simulink model "Bat_SPM"  (R2024a)
settings: Solver=FixedStepAuto  StartTime=0.0  StopTime=t_end  FixedStep=dt  MaxStep=dt  RelTol=1e-3  EnableMultiTasking=on
values from neighbouring files (symbols this model uses):
  I = squeeze(out.I.Data)./4.6    [PI_init.m]
  P0 = 4.1374e3    (= 4137.4)    [PI_init.m]
  Params_P = [sig0,P_atm,E,alpha_cell,Tamb,L,Vh0,A_surf,m_an,xSEI0,MC6,R,A1,B1,     C1,A2,B2,C2,yEC,yDMC]    [PI_init.m]
  V_min = 0    [PI_init.m]
libraries: slpidlib x1
settings Model: Creator=imanebrahimi  LastModifiedBy=imanebrahimi
settings SolverCC: AutoInsertRateTranBlk=on
settings OptimizationCC: DefaultParameterBehavior=Inlined  InlineInvariantSignals=on  EnhancedBackFolding=on  PassReuseOutputArgsAs=Individual arguments  StateBitsets=on  DataBitsets=on  ZeroExternalMemoryAtStartup=off  ZeroInternalMemoryAtStartup=off  NoFixptDivByZeroProtection=on  LifeSpan=1  OptimizeBlockOrder=speed  DifferentSizesBufferReuse=on  EfficientTunableParamExpr=on
settings DebuggingCC: ParameterTunabilityLossMsg=error
settings HardwareCC: ProdBitPerPointer=32  ProdBitPerSizeT=32  ProdBitPerPtrDiffT=32  ProdLargestAtomicFloat=None  ProdIntDivRoundTo=Floor  ProdWordSize=32  ProdHWDeviceType=Generic->Custom
settings SFSimCC: MATLABDynamicMemAlloc=off
settings RTWCC: Description=Embedded Coder  SystemTargetFile=ert.tlc  TLCOptions=-p0  GenCodeOnly=on  TemplateMakefile=ert_default_tmf  GenerateReport=on  RTWVerbose=off  IncludeHyperlinkInReport=on  LaunchReport=on  GPUComputeCapability=3.5
settings CodeAppCC: ForceParamTrailComments=on  IgnoreCustomStorageClasses=off  OperatorAnnotations=on  SimulinkDataObjDesc=on  SFDataObjDesc=on  CustomSymbolStrGlobalVar=rt$N$M  CustomSymbolStrType=$N$M  CustomSymbolStrFcn=$N$M$F  CustomSymbolStrMacro=$N$M  InsertBlockDesc=on
settings ERTTargetCC: TargetLangStandard=C99 (ISO)  CodeReplacementLibrary=ISO_C  GenerateSampleERTMain=on  IncludeMdlTerminateFcn=off  SuppressErrorStatus=on  SupportAbsoluteTime=off  PurelyIntegerCode=on  SupportNonFinite=off  SupportComplex=off  InlinedParameterPlacement=NonHierarchical  RootIOFormat=Structure reference  ERTCustomFileTemplate=example_file_process.tlc

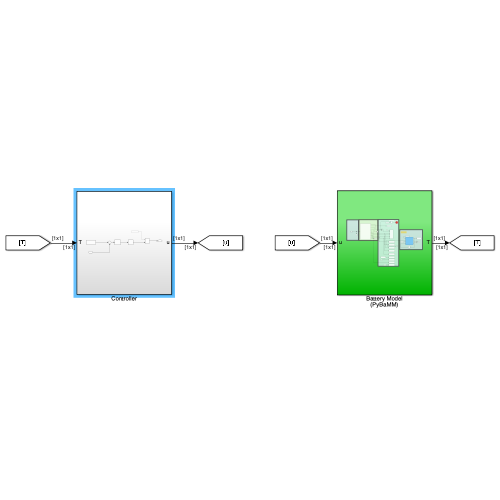
[thumbnail: Simulink's stored preview of the top-level diagram]
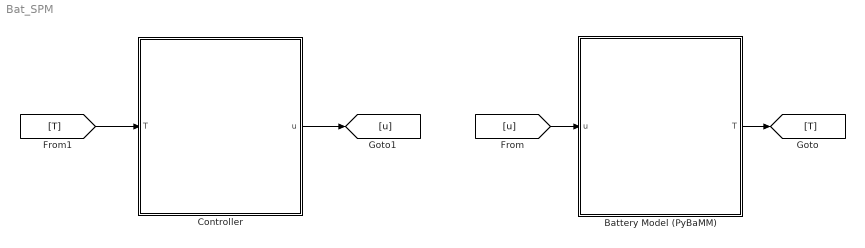
== system Bat_SPM ==
  Battery Model (PyBaMM) : Subsystem
  Controller : Subsystem
  wires:
  [u] -> Battery Model (PyBaMM)/1(u)
  [T] -> Controller/1(T)
  Controller/1(u) -> [u]
  Battery Model (PyBaMM)/1(T) -> [T]

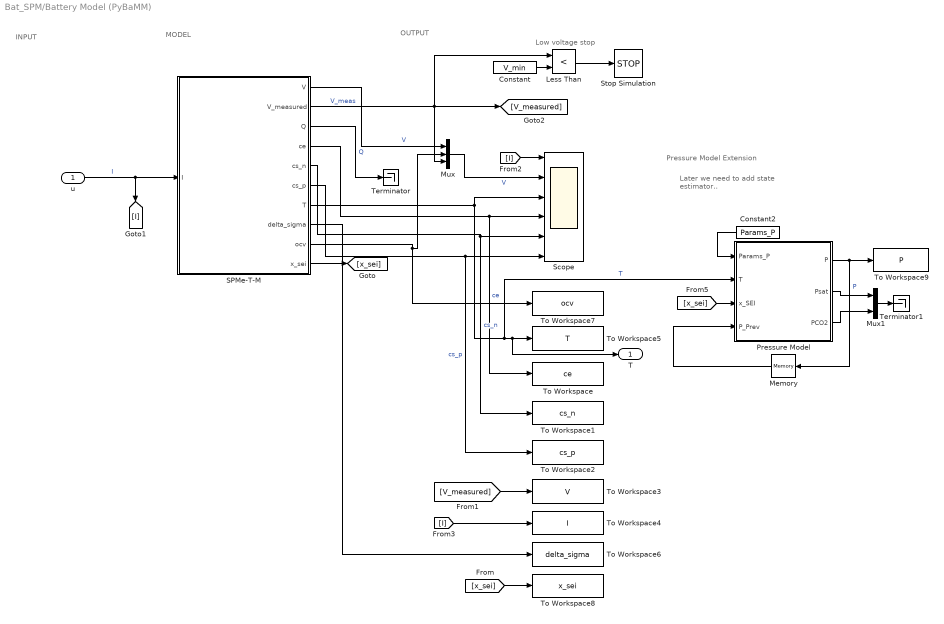
== system Bat_SPM/Battery Model (PyBaMM) ==
  note: INPUT
  note: Low voltage stop
  note: OUTPUT
  note: MODEL
  note: Later we need to add state estimator..
  note: Pressure Model Extension
  u : Inport
  Constant : Constant  Value=V_min
  Constant2 : Constant  Value=Params_P
  Less Than : RelationalOperator  Operator=<  OutDataTypeStr=boolean  RndMeth=Simplest  InputSameDT=off
  Memory : Memory  InitialCondition=P0  InheritSampleTime=on  LinearizeAsDelay=on
  Mux : Mux  Inputs=3
  Mux1 : Mux  Inputs=2
  Pressure Model : MATLAB Function  TreatAsAtomicUnit=on
  SPMe-T-M : Subsystem
  Scope : Scope  NumInputPorts=6
  Stop Simulation : Stop
  Terminator : Terminator
  Terminator1 : Terminator
  To Workspace : ToWorkspace  VariableName=ce  SaveFormat=Timeseries  SampleTime=-1
  To Workspace1 : ToWorkspace  VariableName=cs_n  SaveFormat=Timeseries  SampleTime=-1
  To Workspace2 : ToWorkspace  VariableName=cs_p  SaveFormat=Timeseries  SampleTime=-1
  To Workspace3 : ToWorkspace  VariableName=V  SaveFormat=Timeseries  SampleTime=-1
  To Workspace4 : ToWorkspace  VariableName=I  SaveFormat=Timeseries  SampleTime=-1
  To Workspace5 : ToWorkspace  VariableName=T  SaveFormat=Timeseries  SampleTime=-1
  To Workspace6 : ToWorkspace  VariableName=delta_sigma  SaveFormat=Timeseries  SampleTime=-1
  To Workspace7 : ToWorkspace  VariableName=ocv  SaveFormat=Timeseries  SampleTime=-1
  To Workspace8 : ToWorkspace  VariableName=x_sei  SaveFormat=Timeseries  SampleTime=-1
  To Workspace9 : ToWorkspace  VariableName=P  SaveFormat=Timeseries  SampleTime=-1
  T : Outport
  wires:
  SPMe-T-M/2(V_measured) -> Less Than/1, Mux/3, [V_measured]  "V_meas"
  [V_measured] -> To Workspace3/1
  SPMe-T-M/6(cs_p) -> To Workspace2/1, Scope/6  "cs_p"
  Mux/1 -> Scope/2  "V"
  Less Than/1 -> Stop Simulation/1
  [I] -> Scope/1
  SPMe-T-M/5(cs_n) -> To Workspace1/1, Scope/5  "cs_n"
  Constant/1 -> Less Than/2
  [I] -> To Workspace4/1
  SPMe-T-M/9(ocv) -> Mux/2, To Workspace7/1
  SPMe-T-M/3(Q) -> Terminator/1  "Q"
  SPMe-T-M/1(V) -> Mux/1  "V"
  u/1 -> SPMe-T-M/1(I), [I]  "I"
  SPMe-T-M/8(delta_sigma) -> To Workspace6/1
  SPMe-T-M/7(T) -> Pressure Model/2(T), T/1, To Workspace5/1, Scope/3  "T"
  SPMe-T-M/4(ce) -> To Workspace/1, Scope/4  "ce"
  SPMe-T-M/10(x_sei) -> [x_sei]
  [x_sei] -> To Workspace8/1
  Pressure Model/2(Psat) -> Mux1/1
  Mux1/1 -> Terminator1/1
  Pressure Model/3(PCO2) -> Mux1/2
  Pressure Model/1(P) -> To Workspace9/1, Memory/1  "P"
  Memory/1 -> Pressure Model/4(P_Prev)
  Constant2/1 -> Pressure Model/1(Params_P)
  [x_sei] -> Pressure Model/3(x_SEI)

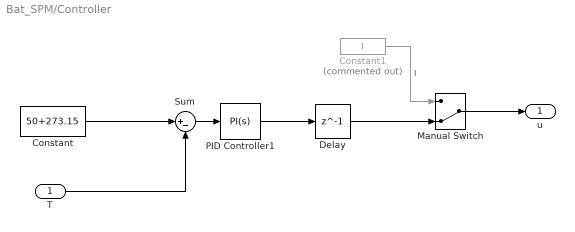
== system Bat_SPM/Controller ==
  T : Inport
  Constant : Constant  Value=50+273.15
  Constant1 : Constant  Commented=on  Value=I
  Delay : Delay  DelayLength=1
  Manual Switch : ManualSwitch  CurrentSetting=0
  PID Controller1 : slpidlib/PID Controller  Controller=PI  Form=Parallel  TimeDomain=Continuous-time  UseExternalTs=off  SampleTime=-1  IntegratorMethod=Forward Euler  FilterMethod=Forward Euler  ControllerParametersSource=internal  P=7.95363343093835  I=0.0486588718627495  UseKiTs=off  D=0  UseExternalDerivativeSource=off  N=100  UseFilter=on  TunerSelectOption=Transfer Function Based (PID Tuner App)  InitialConditionSource=internal  InitialConditionForIntegrator=0  InitialConditionForFilter=0  DifferentiatorICPrevScaledInput=0  ExternalReset=none  TrackingMode=off  Kt=1  LimitOutput=off  SatLimitsSource=internal  UpperSaturationLimit=46  LowerSaturationLimit=0  LinearizeAsGain=on  AntiWindupMode=none  Kb=1  LimitIntegrator=off  UpperIntegratorSaturationLimit=inf  LowerIntegratorSaturationLimit=-inf  POutMin=[]  POutMax=[]  IOutMin=[]  IOutMax=[]  DOutMin=[]  DOutMax=[]  NOutMin=[]  NOutMax=[]  SumOutMin=[]  SumOutMax=[]  SaturationOutMin=[]  SaturationOutMax=[]  PParamMin=[]  PParamMax=[]  IParamMin=[]  IParamMax=[]  DParamMin=[]  DParamMax=[]  NParamMin=[]  NParamMax=[]  KbParamMin=[]  KbParamMax=[]  KtParamMin=[]  KtParamMax=[]  KbOutMin=[]  KbOutMax=[]  KtOutMin=[]  KtOutMax=[]  IntegratorOutMin=[]  IntegratorOutMax=[]  FilterOutMin=[]  FilterOutMax=[]  SumI1OutMin=[]  SumI1OutMax=[]  SumI2OutMin=[]  SumI2OutMax=[]  SumI3OutMin=[]  SumI3OutMax=[]  SumI4OutMin=[]  SumI4OutMax=[]  SumDOutMin=[]  SumDOutMax=[]  DifferentiatorOutMin=[]  DifferentiatorOutMax=[]  FilterDiffOutCoefMin=[]  FilterDiffOutCoefMax=[]  ReciprocalOutMin=[]  ReciprocalOutMax=[]  SumDenOutMin=[]  SumDenOutMax=[]  SumNumOutMin=[]  SumNumOutMax=[]  DivideOutMin=[]  DivideOutMax=[]  UdiffTsProdOutMin=[]  UdiffTsProdOutMax=[]  NTsProdOutMin=[]  NTsProdOutMax=[]  UintegralTsProdOutMin=[]  UintegralTsProdOutMax=[]  UngainTsProdOutMin=[]  UngainTsProdOutMax=[]  ClampingZeroOutDataTypeStr=Inherit: Inherit via back propagation  ClampingZeroOutMin=[]  ClampingZeroOutMax=[]  FilterDenConstantOutDataTypeStr=Inherit: Inherit via back propagation  FilterDenConstantOutMin=[]  FilterDenConstantOutMax=[]  PCopyOutDataTypeStr=Inherit: Inherit via back propagation  PCopyOutMin=[]  PCopyOutMax=[]  NCopyOutDataTypeStr=Inherit: Inherit via back propagation  NCopyOutMin=[]  NCopyOutMax=[]  IntegratorContinuousStateAttributes=''  IntegratorStateMustResolveToSignalObject=off  IntegratorRTWStateStorageClass=Auto  FilterContinuousStateAttributes=''  FilterStateMustResolveToSignalObject=off  FilterRTWStateStorageClass=Auto  ParallelPVariant=InternalParameters  IdealPVariant=Disabled  IVariant=InternalParameters  DVariant=Disabled  IntegratorVariant=Continuous  SatVariant=Disabled  AWVariant=Passthrough  PCopyVariant=Disabled  TRVariant=Disabled  FdbkBlocksVariant=Forward  IdealPFdbkVariant=Disabled  SatFdbkVariant=Disabled  DerivativeFilterVariant=Disabled  NVariant=Disabled  NCopyVariant=Disabled_SignalSpec  FilterICVariant=Disabled  IntegratorICVariant=InternalICs  ExternalResetVariant=Disabled  TRSumVariant=Passthrough  SumFdbkVariant=Disabled  SumVariant=Sum_PI  TsampFilterVariant=InternalTs  TsampNgainVariant=Passthrough  TsampIntegralVariant=Disabled_SignalSpec  ExternalSaturationOutDataTypeStr=Inherit: Same as second input  DerivativeSourceVariant=Disabled
  Sum : Sum  Inputs=|+-
  u : Outport
  wires:
  Manual Switch/1 -> u/1
  Sum/1 -> PID Controller1/1
  PID Controller1/1 -> Delay/1
  Constant/1 -> Sum/1
  Constant1/1 -> Manual Switch/1  "I"
  Delay/1 -> Manual Switch/2
  T/1 -> Sum/2

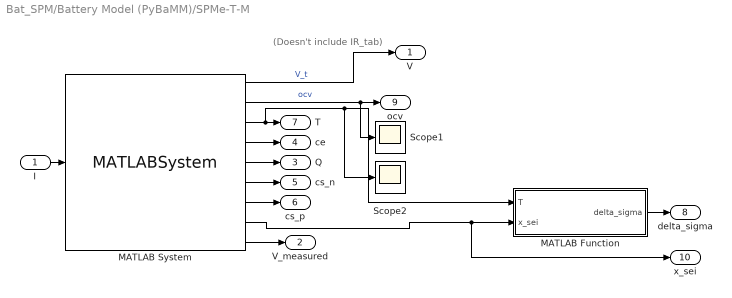
== system Bat_SPM/Battery Model (PyBaMM)/SPMe-T-M ==
  note: (Doesn't include IR_tab)
  I : Inport
  MATLAB Function : MATLAB Function  TreatAsAtomicUnit=on
  MATLAB System : MATLABSystem  System=pybamm_bat  SimulateUsing=Interpreted execution
      mask Type: pybamm_bat
      mask Display:
      | disp('pybamm_bat');
      | port_label('input',1,'current');
      | port_label('output',1,'V_t');
      | port_label('output',2,'ocv');
      | port_label('output',3,'T');
      | port_label('output',4,'ce');
      | port_label('output',5,'heating');
      | port_label('output',6,'neg_conc');
      | port_label('output',7,'pos_conc');
      | port_label('output',8,'x_sei');
      | port_label('output',9,'V_meas');
  Scope1 : Scope
  Scope2 : Scope
  V : Outport
  V_measured : Outport  Port=2
  Q : Outport  Port=3  VectorParamsAs1DForOutWhenUnconnected=off
  ce : Outport  Port=4
  cs_n : Outport  Port=5  VectorParamsAs1DForOutWhenUnconnected=off
  cs_p : Outport  Port=6  VectorParamsAs1DForOutWhenUnconnected=off
  T : Outport  Port=7
  delta_sigma : Outport  Port=8
  ocv : Outport  Port=9
  x_sei : Outport  Port=10
  wires:
  MATLAB System/4 -> ce/1
  MATLAB System/5 -> Q/1
  MATLAB System/6 -> cs_n/1
  MATLAB System/7 -> cs_p/1
  MATLAB System/1 -> V/1  "V_t"
  MATLAB System/9 -> V_measured/1
  MATLAB System/2 -> Scope1/1, ocv/1  "ocv"
  I/1 -> MATLAB System/1
  MATLAB System/3 -> MATLAB Function/1(T), Scope2/1, T/1
  MATLAB System/8 -> x_sei/1, MATLAB Function/2(x_sei)
  MATLAB Function/1(delta_sigma) -> delta_sigma/1

== matlab function Bat_SPM/Battery Model (PyBaMM)/SPMe-T-M/MATLAB Function ==
  data: T input; x_sei input; delta_sigma output
function delta_sigma  = expansion(T,x_sei)
%XSEI2PTOTAL 
% Mechanical params
M_C6 = 72/1000; %kg/mol
% V_head_0 = 6.65e-6; %m3 (0.121*0.074*0.0055)*0.135
% L = 2.4/1000; %m
% E = 0.19e6; %Pa
% alpha_cell = 1.1e-6; %m/K
% P_atm = 101; %kPa
% P_crit = 158.7731; %kPa
R = 8.3145; %J.mol-1.K-1
A = 0.009; %m2 (0.121*0.074)
DMC = [6.4338; 1413; -44.25]; %Antoine coeffs [A B C] 
EC = [6.4897; 1836.57; -102.23];
y_dmc = 0.7;
y_ec = 1-y_dmc;         
m_an = 0.0191; 
x_sei_0 = 0.15;
% T_amb = 273.15+25; % K
% sigma_0 = 1.5120e+04;

% Internal cell pressure
V_head_0 = 6.65e-06; %m-3
L_p0 = 2.4e-3; %m for 2 poron
E_p = 0.19e6; %Pa Young's modulus for poron
% E_c = 1e12; %assume large by default
alpha = 1.1e-6; %m/K
P_atm = 101e3; %Pa
% P_crit = 158e3; %Pa
% P0 = 14e3; %Pa
R = 8.3145; %J.mol-1.K-1
% k_b = 1.380649e-23; %m2.kg.s-2.K-1;
T_amb = 273.15+25; % K
sigma_0 = 1.5120e+04;
% L_cs0 = 5.5e-3; %m initial cell solid thickness
% V_cell = 0.130*0.089*0.055; % [130mm×89mm×5.5mm] active material

% P_elyte
Psat_EC = 10.^(EC(1)-EC(2)./(EC(3)+T));
Psat_DMC = 10.^(DMC(1)-DMC(2)./(DMC(3)+T)); 
P_elyte = (y_dmc*Psat_DMC + y_ec*Psat_EC)*1e3; 

% P_CO2
n_CO2 = 0.5*m_an/M_C6*(x_sei_0-x_sei);

% Solve for gas volume and pressure
delta_sigma_calc = P_elyte - sigma_0 - P_atm;
a = 1;
b = -(V_head_0 + A.*(L_p0/E_p*(delta_sigma_calc) - alpha.*(T-T_amb)));
c = -A*L_p0/E_p.*n_CO2.*R.*(T);
V_g0 = (-b+sqrt(max(b.^2-4.*a.*c,0)))/(2*a);
V_g = max(V_g0, V_head_0); % min V_g = V_head_0

P_CO2 = n_CO2.*R.*T./V_g;
P_gas = P_elyte + P_CO2;

delta_sigma = max(P_gas-P_atm-sigma_0, E_p./L_p0.*alpha.*(T-T_amb));
end

== matlab function Bat_SPM/Battery Model (PyBaMM)/Pressure Model ==
  data: Params_P input; T input; x_SEI input; P_Prev input; P output; Psat output; PCO2 output
function [P,Psat,PCO2] = Pressure(Params_P,T,x_SEI,P_Prev)

% Parameters
sig0        = Params_P(1);
P_atm       = Params_P(2);
E           = Params_P(3);
alpha_cell  = Params_P(4);
Tamb        = Params_P(5);
L           = Params_P(6);
Vh0         = Params_P(7);
A_surf      = Params_P(8);
m_an        = Params_P(9);
xSEI0       = Params_P(10);
MC6         = Params_P(11);
R           = Params_P(12);
A1          = Params_P(13);
B1          = Params_P(14);
C1          = Params_P(15);
A2          = Params_P(16);
B2          = Params_P(17);
C2          = Params_P(18);
yEC         = Params_P(19);
yDMC        = Params_P(20);

% Pressure (Algebraic) model
d_sigma     = max(P_Prev-sig0-P_atm,E*alpha_cell*(T-Tamb)/L);
dd          = L*d_sigma/E;
Vh          = Vh0+A_surf*(dd-alpha_cell*(T-Tamb));
nCO2        = m_an*(xSEI0-x_SEI)/(2*MC6);                        % [mol]
PCO2        = nCO2*R*T/Vh;                                       % [Pa]
PsatEC      = (10^(A1-B1/(T+C1)))*1e3;                           % [Pa]
PsatDMC     = (10^(A2-B2/(T+C2)))*1e3;                           % [Pa]
Psat        = yEC*PsatEC+yDMC*PsatDMC;                           % [Pa]
P           = PCO2+Psat;                                         % [Pa]
